simulink model "Control_systemR2024a"  (R2025b)
settings: Solver=FixedStepAuto  StartTime=0.0  StopTime=5  FixedStep=0.01  RelTol=1e-3
values from neighbouring files (symbols this model uses):
  beta = [beta1, beta2, beta3, beta4]    [initialize_simulink.m]
  calMp = Adgsl10m1' * calM1 * Adgsl10m1    [initialize_simulink.m]
  lM = zeros(4)    [initialize_simulink.m]
  m4g = m4 * 9.81    (= 68.67)    [initialize_simulink.m]
  xi = [xi1, xi2, xi3, xi4]    [initialize_simulink.m]
settings Model: Creator=81135  LastModifiedBy=dixiao

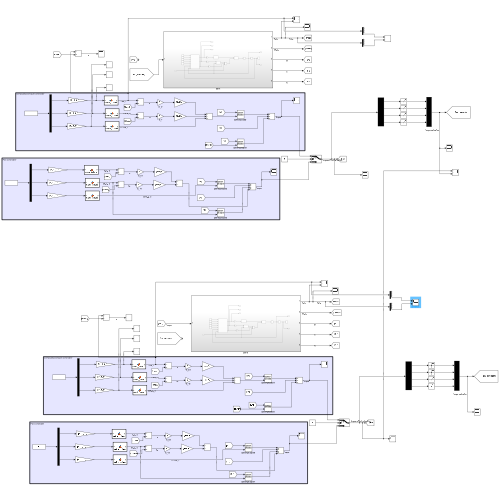
[thumbnail: Simulink's stored preview of the top-level diagram]
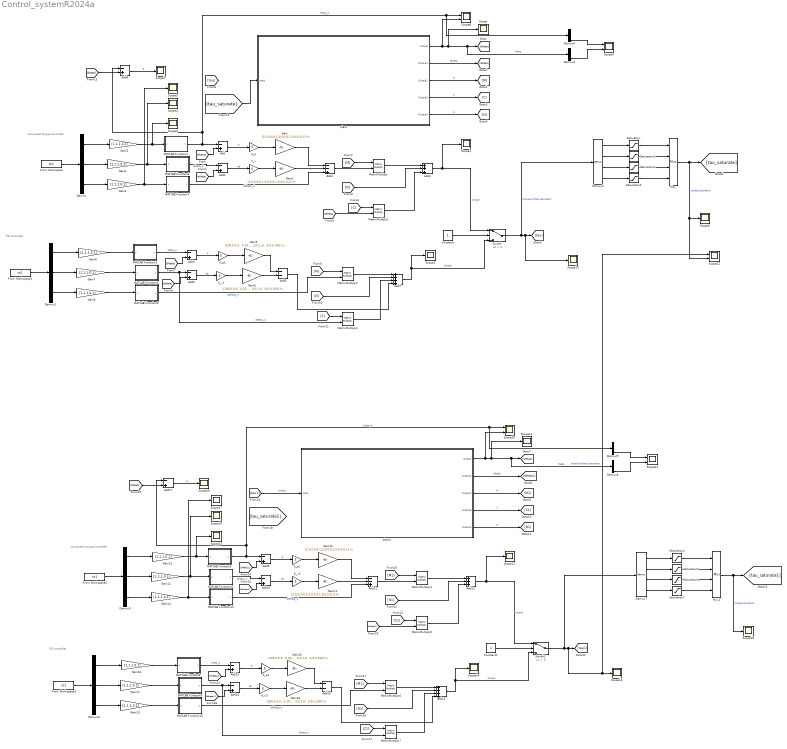
== system Control_systemR2024a ==
  note: PD controller
  note: computed torque controller
  note: computed torque controller
  note: PD controller
  Add{,1,4..5,8..10,13..14,17} (10 alike) : Sum  Inputs=-+
  Add11 : Sum  Inputs=--+
  Add12 : Sum  Inputs=+++
  Add15 : Sum  Inputs=--
  Add16 : Sum  Inputs=++++
  Add2 : Sum  Inputs=--+
  Add3 : Sum  Inputs=+++
  Add6 : Sum  Inputs=--
  Add7 : Sum  Inputs=++++
  Constant : Constant
  Constant1 : Constant
  Demux{,1,5..6} (4 alike) : Demux  Outputs=3
  Demux{2..4,7..9} (6 alike) : Demux
  From Workspace{,1..3} (4 alike) : FromWorkspace  VariableName=ts1
  Gain{,1,10..11} (4 alike) : Gain  Gain=[1,0,0,0;0,1,0,0;0,0,1,0;0,0,0,1]  Multiplication=Matrix(K*u)
  Gain{2..4,7..9,12..14,17..19} (12 alike) : Gain  Gain=[1,1,1,0.1]
  Gain{5..6,15..16} (4 alike) : Gain  Gain="[100,0,0,0;  0,100,0,0;  0,0,1,0;  0,0,0,100]"  Multiplication=Matrix(K*u)
  K_p{,1..3} (4 alike) : Gain  Gain=5
  K_v{,1..3} (4 alike) : Gain  Gain=5
  MATLAB Function1 : MATLAB Function  TreatAsAtomicUnit=on
  MATLAB Function10 : MATLAB Function  TreatAsAtomicUnit=on
  MATLAB Function11 : MATLAB Function  TreatAsAtomicUnit=on
  MATLAB Function12 : MATLAB Function  TreatAsAtomicUnit=on
  MATLAB Function2 : MATLAB Function  TreatAsAtomicUnit=on
  MATLAB Function3 : MATLAB Function  TreatAsAtomicUnit=on
  MATLAB Function4 : MATLAB Function  TreatAsAtomicUnit=on
  MATLAB Function5 : MATLAB Function  TreatAsAtomicUnit=on
  MATLAB Function6 : MATLAB Function  TreatAsAtomicUnit=on
  MATLAB Function7 : MATLAB Function  TreatAsAtomicUnit=on
  MATLAB Function8 : MATLAB Function  TreatAsAtomicUnit=on
  MATLAB Function9 : MATLAB Function  TreatAsAtomicUnit=on
  MatrixMultiply{,1..7} (8 alike) : Product  Multiplication=Matrix(*)
  Mux : Mux
  Mux1 : Mux
  Saturation : Saturate  UpperLimit=2000  LowerLimit=-2000
  Saturation{1..2,5..6} (4 alike) : Saturate  UpperLimit=1000  LowerLimit=-1000
  Saturation3 : Saturate  UpperLimit=100  LowerLimit=-100
  Saturation4 : Saturate  UpperLimit=2000  LowerLimit=-2000
  Saturation7 : Saturate  UpperLimit=100  LowerLimit=-100
  Scope{,1..7,10..19} (18 alike) : Scope
      Scope settings: ActiveDisplayYMinimum=-0.45551  ActiveDisplayYMaximum=2.83276
      Scope1 settings: ActiveDisplayYMinimum=-5169.19127  ActiveDisplayYMaximum=5422.5513  DataLoggingVariableName=ScopeData3
      Scope10 settings: ActiveDisplayYMinimum=-2408.79583  ActiveDisplayYMaximum=5518.79264  DataLoggingVariableName=ScopeData4
      Scope11 settings: ActiveDisplayYMinimum=-0.45551  ActiveDisplayYMaximum=2.83276  DataLoggingVariableName=ScopeData5
      Scope12 settings: ActiveDisplayYMinimum=-5169.19127  ActiveDisplayYMaximum=5422.5513  DataLoggingVariableName=ScopeData6
      Scope13 settings: ActiveDisplayYMinimum=-5240.02366  ActiveDisplayYMaximum=5364.1419  DataLoggingVariableName=ScopeData7
      Scope14 settings: ActiveDisplayYMinimum=-5091.129  ActiveDisplayYMaximum=5351.713  DataLoggingVariableName=ScopeData8
      Scope15 settings: ActiveDisplayYMinimum=-0.125  ActiveDisplayYMaximum=1.125  DataLoggingVariableName=ScopeData9
      Scope16 settings: ActiveDisplayYMinimum=-0.41667  ActiveDisplayYMaximum=3.75  DataLoggingVariableName=ScopeData10
      Scope17 settings: ActiveDisplayYMinimum=-41.66667  ActiveDisplayYMaximum=41.66667  DataLoggingVariableName=ScopeData11
      Scope18 settings: ActiveDisplayYMinimum=-2500  ActiveDisplayYMaximum=2500  DataLoggingVariableName=ScopeData12
      Scope19 settings: ActiveDisplayYMinimum=-0.0046  ActiveDisplayYMaximum=0.04138  DataLoggingVariableName=ScopeData13
      Scope2 settings: ActiveDisplayYMinimum=-5091.129  ActiveDisplayYMaximum=5351.713  DataLoggingVariableName=ScopeData2
      Scope3 settings: ActiveDisplayYMinimum=-0.125  ActiveDisplayYMaximum=1.125  DataLoggingVariableName=ScopeData4
      Scope4 settings: ActiveDisplayYMinimum=-0.41667  ActiveDisplayYMaximum=3.75  DataLoggingVariableName=ScopeData5
      Scope5 settings: ActiveDisplayYMinimum=-41.66667  ActiveDisplayYMaximum=41.66667  DataLoggingVariableName=ScopeData6
      Scope6 settings: ActiveDisplayYMinimum=-2500  ActiveDisplayYMaximum=2500  DataLoggingVariableName=ScopeData7
      Scope7 settings: ActiveDisplayYMinimum=-1.1474  ActiveDisplayYMaximum=1.79852
  Scope{8..9,20..22} (5 alike) : Scope  NumInputPorts=2
      Scope20 settings: ActiveDisplayYMinimum=-0.1296  ActiveDisplayYMaximum=1.16638  DataLoggingVariableName=ScopeData14
      Scope21 settings: ActiveDisplayYMinimum=-0.01253  ActiveDisplayYMaximum=0.11281  DataLoggingVariableName=ScopeData15
      Scope22 settings: ActiveDisplayYMinimum=1.92293  ActiveDisplayYMaximum=75.33497  DataLoggingVariableName=ScopeData16
      Scope8 settings: ActiveDisplayYMinimum=-1.3690570459134255  ActiveDisplayYMaximum=2.8522624254214288  DataLoggingVariableName=ScopeData2
      Scope9 settings: ActiveDisplayYMinimum=-0.01253  ActiveDisplayYMaximum=0.11281  DataLoggingVariableName=ScopeData3
  Switch : Switch  Criteria=u2 > Threshold  SaturateOnIntegerOverflow=off  InputSameDT=off
  Switch1 : Switch  Criteria=u2 > Threshold  SaturateOnIntegerOverflow=off  InputSameDT=off
  plant : Subsystem
  plant1 : Subsystem
  wires:
  plant/1(Output) -> Scope8/2, Demux3/1, [theta], Scope/1  "theta"
  plant/2(Output1) -> [dtheta]  "dtheta"
  plant/3(Output2) -> [M]  "M"
  plant/4(Output3) -> [C]  "C"
  plant/5(Output4) -> [N]  "N"
  Add/1 -> K_p/1  "e"
  [dtheta] -> MatrixMultiply1/2
  MatrixMultiply/1 -> Add3/1
  Gain1/1 -> Add2/2
  Demux/2 -> Gain2/1
  [N] -> Add3/2
  From Workspace/1 -> Demux/1
  [theta] -> Add/2
  Add1/1 -> K_v/1  "de"
  MATLAB Function6/1(y) -> Add1/1  "dtheta_d"
  [M] -> MatrixMultiply/1
  [dtheta] -> Add1/2
  Add3/1 -> Switch/1, Scope1/1  "torque"
  [C] -> MatrixMultiply1/1
  Add2/1 -> MatrixMultiply/2
  MATLAB Function7/1(y) -> Add2/3  "ddtheta_d"
  MatrixMultiply1/1 -> Add3/3
  Gain/1 -> Add2/1
  Demux/1 -> Gain3/1
  MATLAB Function1/1(y) -> Demux4/1, Scope8/1, Add8/1, Add/1  "theta_d"
  Gain4/1 -> Scope5/1, MATLAB Function7/1(u)
  Gain2/1 -> Scope4/1, MATLAB Function6/1(u)
  Gain3/1 -> Scope3/1, MATLAB Function1/1(u)
  K_v/1 -> Gain1/1
  K_p/1 -> Gain/1
  Demux/3 -> Gain4/1
  [N] -> Add7/2
  Demux1/2 -> Gain7/1
  Gain6/1 -> Add6/2
  Add4/1 -> K_p1/1  "e"
  [C] -> MatrixMultiply3/1
  Add7/1 -> Switch/3, Scope2/1  "torque"
  MatrixMultiply3/1 -> Add7/3
  Gain5/1 -> Add6/1
  MATLAB Function4/1(y) -> MatrixMultiply2/2  "ddtheta_d"
  Demux1/1 -> Gain8/1
  Gain9/1 -> MATLAB Function4/1(u)
  Gain8/1 -> MATLAB Function2/1(u)
  Gain7/1 -> MATLAB Function3/1(u)
  MATLAB Function2/1(y) -> Add4/1  "theta_d"
  From Workspace1/1 -> Demux1/1
  MatrixMultiply2/1 -> Add7/1
  Demux1/3 -> Gain9/1
  K_v1/1 -> Gain6/1
  [M] -> MatrixMultiply2/1
  MATLAB Function3/1(y) -> MatrixMultiply3/2, Add5/1  "dtheta_d"
  [dtheta] -> Add5/2
  Add5/1 -> K_v1/1  "de"
  K_p1/1 -> Gain5/1
  [theta] -> Add4/2
  Add6/1 -> Add7/4
  Constant/1 -> Switch/2
  Demux2/4 -> Saturation3/1
  Demux2/2 -> Saturation1/1
  Demux2/1 -> Saturation/1
  Demux2/3 -> Saturation2/1
  Switch/1 -> Demux2/1, Scope10/1, [tau]  "torque without saturation"
  Saturation/1 -> Mux/1
  Saturation1/1 -> Mux/2
  Saturation2/1 -> Mux/3
  Saturation3/1 -> Mux/4
  Mux/1 -> Scope22/2, Scope6/1, [tau_saturate]  "torque saturation"
  [theta] -> Add8/2
  Add8/1 -> Scope7/1  "e"
  Demux4/4 -> Scope9/1
  Demux3/4 -> Scope9/2
  [theta1] -> Add17/2
  Add17/1 -> Scope19/1  "e"
  Demux9/4 -> Scope21/1
  Saturation6/1 -> Mux1/3
  Add9/1 -> K_p2/1  "e"
  Gain16/1 -> Add15/2
  Saturation5/1 -> Mux1/2
  MATLAB Function5/1(y) -> Demux9/1, Scope20/1, Add17/1, Add9/1  "theta_d"
  [C1] -> MatrixMultiply7/1
  Gain17/1 -> MATLAB Function9/1(u)
  MATLAB Function10/1(y) -> MatrixMultiply6/2  "ddtheta_d"
  Saturation4/1 -> Mux1/1
  Switch1/1 -> Demux7/1, Scope22/1, Scope13/1, [tau1]  "torque without saturation"
  Mux1/1 -> Scope18/1, [tau_saturate1]  "torque saturation"
  Saturation7/1 -> Mux1/4
  MATLAB Function12/1(y) -> Add11/3  "ddtheta_d"
  [dtheta1] -> Add10/2
  MATLAB Function8/1(y) -> Add13/1  "theta_d"
  [theta1] -> Add9/2
  plant1/3(Output2) -> [M1]  "M"
  [dtheta1] -> Add14/2
  plant1/2(Output1) -> [dtheta1]  "dtheta"
  Demux7/1 -> Saturation4/1
  MatrixMultiply6/1 -> Add16/1
  Gain10/1 -> Add11/1
  Demux6/1 -> Gain18/1
  From Workspace2/1 -> Demux5/1
  Add15/1 -> Add16/4
  K_p3/1 -> Gain15/1
  Gain15/1 -> Add15/1
  [M1] -> MatrixMultiply6/1
  Demux6/3 -> Gain19/1
  plant1/1(Output) -> Scope20/2, Demux8/1, [theta1], Scope11/1  "theta"
  Add14/1 -> K_v3/1  "de"
  K_v2/1 -> Gain11/1
  MatrixMultiply7/1 -> Add16/3
  Demux8/4 -> Scope21/2
  K_v3/1 -> Gain16/1
  [N1] -> Add16/2
  Demux5/3 -> Gain14/1
  Gain12/1 -> Scope16/1, MATLAB Function11/1(u)
  [dtheta1] -> MatrixMultiply5/2
  [tau1] -> plant1/1(Input)  "torque"
  Constant1/1 -> Switch1/2
  K_p2/1 -> Gain10/1
  Gain19/1 -> MATLAB Function10/1(u)
  Gain13/1 -> Scope15/1, MATLAB Function5/1(u)
  plant1/4(Output3) -> [C1]  "C"
  Demux7/4 -> Saturation7/1
  Add16/1 -> Switch1/3, Scope14/1  "torque"
  MatrixMultiply4/1 -> Add12/1
  MATLAB Function11/1(y) -> Add10/1  "dtheta_d"
  Add12/1 -> Switch1/1, Scope12/1  "torque"
  Demux5/2 -> Gain12/1
  [C1] -> MatrixMultiply5/1
  Gain18/1 -> MATLAB Function8/1(u)
  [M1] -> MatrixMultiply4/1
  Demux5/1 -> Gain13/1
  MATLAB Function9/1(y) -> MatrixMultiply7/2, Add14/1  "dtheta_d"
  From Workspace3/1 -> Demux6/1
  [theta1] -> Add13/2
  Add10/1 -> K_v2/1  "de"
  MatrixMultiply5/1 -> Add12/3
  Demux7/2 -> Saturation5/1
  Add11/1 -> MatrixMultiply4/2
  Gain14/1 -> Scope17/1, MATLAB Function12/1(u)
  Demux7/3 -> Saturation6/1
  Gain11/1 -> Add11/2
  Demux6/2 -> Gain17/1
  [N1] -> Add12/2
  plant1/5(Output4) -> [N1]  "N"
  Add13/1 -> K_p3/1  "e"
  [tau_saturate] -> plant/1(Input)

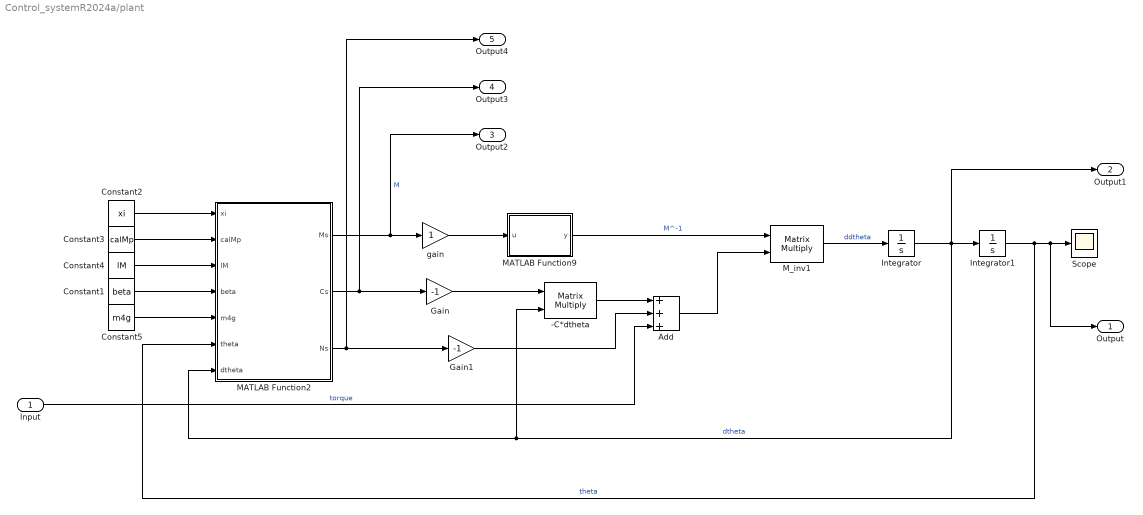
== system Control_systemR2024a/plant ==
  Input : Inport
  -C*dtheta : Product  Multiplication=Matrix(*)
  Add : Sum  Inputs=+++
  Constant1 : Constant  Value=beta
  Constant2 : Constant  Value=xi
  Constant3 : Constant  Value=calMp
  Constant4 : Constant  Value=lM
  Constant5 : Constant  Value=m4g
  Gain : Gain  Gain=-1
  Gain1 : Gain  Gain=-1
  Integrator : Integrator  InitialCondition=[0;0;0;0]
  Integrator1 : Integrator  InitialCondition=[0;0;0;0]
  MATLAB Function2 : MATLAB Function  TreatAsAtomicUnit=on
  MATLAB Function9 : MATLAB Function  TreatAsAtomicUnit=on
  M_inv1 : Product  Multiplication=Matrix(*)
  Scope : Scope
      settings: ActiveDisplayYMinimum=-0.13004  ActiveDisplayYMaximum=1.17037
  gain : Gain
  Output : Outport
  Output1 : Outport  Port=2
  Output2 : Outport  Port=3
  Output3 : Outport  Port=4
  Output4 : Outport  Port=5
  wires:
  MATLAB Function2/1(Ms) -> Output2/1, gain/1  "M"
  Integrator/1 -> Output1/1, -C*dtheta/2, MATLAB Function2/7(dtheta), Integrator1/1  "dtheta"
  Gain/1 -> -C*dtheta/1
  Constant4/1 -> MATLAB Function2/3(lM)
  -C*dtheta/1 -> Add/1
  Constant3/1 -> MATLAB Function2/2(calMp)
  Integrator1/1 -> MATLAB Function2/6(theta), Output/1, Scope/1  "theta"
  M_inv1/1 -> Integrator/1  "ddtheta"
  MATLAB Function2/3(Ns) -> Output4/1, Gain1/1
  Constant1/1 -> MATLAB Function2/4(beta)
  Gain1/1 -> Add/2
  Constant5/1 -> MATLAB Function2/5(m4g)
  gain/1 -> MATLAB Function9/1(u)
  MATLAB Function2/2(Cs) -> Output3/1, Gain/1
  Constant2/1 -> MATLAB Function2/1(xi)
  Add/1 -> M_inv1/2
  MATLAB Function9/1(y) -> M_inv1/1  "M^-1"
  Input/1 -> Add/3  "torque"

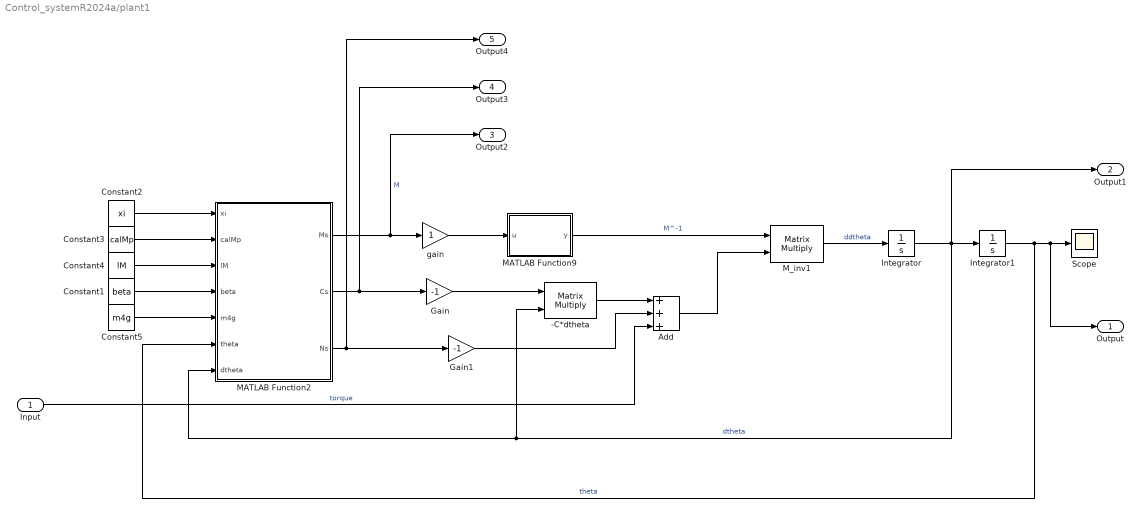
== system Control_systemR2024a/plant1 ==
  Input : Inport
  -C*dtheta : Product  Multiplication=Matrix(*)
  Add : Sum  Inputs=+++
  Constant1 : Constant  Value=beta
  Constant2 : Constant  Value=xi
  Constant3 : Constant  Value=calMp
  Constant4 : Constant  Value=lM
  Constant5 : Constant  Value=m4g
  Gain : Gain  Gain=-1
  Gain1 : Gain  Gain=-1
  Integrator : Integrator  InitialCondition=[0;0;0;0]
  Integrator1 : Integrator  InitialCondition=[0;0;0;0]
  MATLAB Function2 : MATLAB Function  TreatAsAtomicUnit=on
  MATLAB Function9 : MATLAB Function  TreatAsAtomicUnit=on
  M_inv1 : Product  Multiplication=Matrix(*)
  Scope : Scope
      settings: ActiveDisplayYMinimum=-0.13004  ActiveDisplayYMaximum=1.17037
  gain : Gain
  Output : Outport
  Output1 : Outport  Port=2
  Output2 : Outport  Port=3
  Output3 : Outport  Port=4
  Output4 : Outport  Port=5
  wires:
  MATLAB Function2/1(Ms) -> Output2/1, gain/1  "M"
  Integrator/1 -> Output1/1, -C*dtheta/2, MATLAB Function2/7(dtheta), Integrator1/1  "dtheta"
  Gain/1 -> -C*dtheta/1
  Constant4/1 -> MATLAB Function2/3(lM)
  -C*dtheta/1 -> Add/1
  Constant3/1 -> MATLAB Function2/2(calMp)
  Integrator1/1 -> MATLAB Function2/6(theta), Output/1, Scope/1  "theta"
  M_inv1/1 -> Integrator/1  "ddtheta"
  MATLAB Function2/3(Ns) -> Output4/1, Gain1/1
  Constant1/1 -> MATLAB Function2/4(beta)
  Gain1/1 -> Add/2
  Constant5/1 -> MATLAB Function2/5(m4g)
  gain/1 -> MATLAB Function9/1(u)
  MATLAB Function2/2(Cs) -> Output3/1, Gain/1
  Constant2/1 -> MATLAB Function2/1(xi)
  Add/1 -> M_inv1/2
  MATLAB Function9/1(y) -> M_inv1/1  "M^-1"
  Input/1 -> Add/3  "torque"

== matlab function Control_systemR2024a/MATLAB Function5 ==
  data: u input; y output
function y = matrix_column(u)

    y = u(:);
end

== matlab function Control_systemR2024a/MATLAB Function8 ==
  data: u input; y output
function y = matrix_column(u)

    y = u(:);
end

== matlab function Control_systemR2024a/MATLAB Function9 ==
  data: u input; y output
function y = matrix_column(u)

    y = u(:);
end

== matlab function Control_systemR2024a/plant1/MATLAB Function2 ==
  data: xi input; Ms output; calMp input; lM input; beta input; m4g input; theta input; dtheta input; Cs output; Ns output
function [Ms,Cs,Ns] = MCNsim(xi,calMp,lM,beta,m4g,theta,dtheta)
    n = length(theta);
    Ms = zeros(n, n);
    Cs = zeros(n, n);
    % Ns = zeros(n, 1);
    
    % ========== 关键步骤1：预先计算所有需要的变换矩阵 g = exp(ξθ) ==========
    g = cell(1, n+1);
    g{1} = eye(4);
    for i = 1:n
        xi_i = xi(:, i);
        g_joint = expm(hat_se3(xi_i) * theta(i));
        g{i+1} = g{i} * g_joint;
    end
    
    % ========== 关键步骤2：计算所有 A_{ij} ==========
    A = cell(n, n);
    for i = 1:n
        for j = 1:n
            if i > j
                g_ji = inv(g{j+1}) * g{i+1};
                A{i,j} = inv(adjmg(g_ji));
            elseif i == j
                A{i,j} = eye(6);
            else
                A{i,j} = zeros(6);
            end
        end
    end
    
    % ========== 步骤3：计算惯性矩阵 M ==========
    for i = 1:n
        for j = 1:n
            M_ij = 0;
            for l = lM(i, j):n
                M_l = calMp(1:6, 1:6, l);
                term = xi(:, i)' * A{l, i}' * M_l * A{l, j} * xi(:, j);
                M_ij = M_ij + term;
            end
            Ms(i, j) = M_ij;
        end
    end
    
    % ========== 步骤4：计算科氏矩阵 C（解析公式） ==========
    for i = 1:n
        for j = 1:n
            C_ij = 0;
            for k = 1:n
                dM_ij_dtheta_k = compute_partial_M(xi, calMp, lM, A, i, j, k, n);
                dM_ik_dtheta_j = compute_partial_M(xi, calMp, lM, A, i, k, j, n);
                dM_kj_dtheta_i = compute_partial_M(xi, calMp, lM, A, k, j, i, n);
                C_ij = C_ij + 0.5 * (dM_ij_dtheta_k + dM_ik_dtheta_j - dM_kj_dtheta_i) * dtheta(k);
            end
            Cs(i, j) = C_ij;
        end
    end
    
    % ========== 步骤5：计算 N（根据图片公式和你的物理参数） ==========
    % 公式：N_i = ∂V/∂θ_i + β_i * θ̇_i
    
    % 5.1 计算重力势能梯度 ∂V/∂θ_i
    grad_V = compute_gravity_potential_gradient(xi, calMp, g, n);
    
    % 5.2 计算粘性摩擦项 β_i * θ̇_i 
    % 你的beta是向量: [beta1, beta2, beta3, beta4]，单位对应各关节类型
    friction_term = beta(:) .* dtheta(:); % 确保维度匹配
    
    % 5.3 计算总N项: N = ∂V/∂θ + β * θ̇
    Ns = -grad_V + friction_term;
end

% ========== 辅助函数：计算重力势能梯度 ∂V/∂θ (已根据你的代码调整) ==========
function grad_V = compute_gravity_potential_gradient(xi, calMp, g, n)
    % 计算重力势能 V(θ) 关于 θ 的梯度
    % 根据旋量理论：∂V/∂θ_i = Σ_{l=i}^n ξ_i^T * (Ad^{-1}(g_{0l}))^T * M_l * G_0
    % 其中 G_0 是基座标系下的重力旋量
    
    grad_V = zeros(n, 1);
    
    % 基座标系下的重力加速度向量 (沿负z轴，大小9.81 m/s²)
    % 注意：重力对旋量的贡献取决于表示法
    % 对于空间旋量 ξ = [v; ω]，重力旋量为 G = [0; -g]
    g_accel = [0; 0; -9.81]; % 重力加速度向量
    
    % 构造基座标系下的重力旋量 G_0
    % 根据你的旋量构造方式 (xi = [-hat(w)*q; w])，这是空间旋量表示
    % 对于空间旋量，重力只有线速度部分：G_0 = [-g_accel; 0]
    G_base = zeros(6, 1);
    G_base(1:3) = -g_accel; % 线速度部分：负重力加速度
    G_base(4:6) = zeros(3,1); % 角速度部分：0
    
    for i = 1:n
        sum_term = 0;
        for l = i:n
            % 连杆 l 的空间惯性矩阵 (已在空间坐标系下，通过伴随变换得到)
            M_l = calMp(1:6, 1:6, l);
            
            % 从基座到连杆 l 的变换矩阵 g_{0l}
            g_0l = g{l+1};
            
            % 计算 Ad^{-1}(g_{0l}) 的转置
            Ad_inv = inv(adjmg(g_0l));
            Ad_inv_T = Ad_inv';
            
            % 计算该项对梯度 ∂V/∂θ_i 的贡献
            % 根据旋量理论，这是重力在关节i方向产生的广义力
            contribution = xi(:, i)' * Ad_inv_T * M_l * G_base;
            sum_term = sum_term + contribution;
        end
        
        % 得到的 sum_term 实际上是重力矩 G_i = -∂V/∂θ_i
        % 因此势能梯度为 ∂V/∂θ_i = -sum_term
        grad_V(i) = -sum_term;
    end
end

% ========== 其他辅助函数保持不变 ==========
function dM_ij_dtheta_k = compute_partial_M(xi, calMp, lM, A, i, j, k, n)
    dM_ij_dtheta_k = 0;
    
    for l = lM(i, j):n
        M_l = calMp(1:6, 1:6, l);
        xi_i = xi(:, i);
        xi_j = xi(:, j);
        xi_k = xi(:, k);
        
        if k <= l
            % 计算 ad(A_{ki} * xi_i)
            A_ki_xi_i = A{k, i} * xi_i;
            ad_Aki_xi_i = adjoint_lie_algebra(A_ki_xi_i);
            
            % 计算 ad(A_{kj} * xi_j)
            A_kj_xi_j = A{k, j} * xi_j;
            ad_Akj_xi_j = adjoint_lie_algebra(A_kj_xi_j);
            
            term1 = (ad_Aki_xi_i * xi_k)' * A{l, k}' * M_l * A{l, j} * xi_j;
            term2 = xi_i' * A{l, i}' * M_l * A{l, k} * (ad_Akj_xi_j * xi_k);
            
            dM_ij_dtheta_k = dM_ij_dtheta_k + term1 + term2;
        end
    end
end

function ad_xi = adjoint_lie_algebra(xi)
    v = xi(1:3);
    w = xi(4:6);
    w_hat = hatm_num(w);
    v_hat = hatm_num(v);
    ad_xi = [w_hat, v_hat;
             zeros(3), w_hat];
end

function se3 = hat_se3(xi)
    v = xi(1:3);
    w = xi(4:6);
    se3 = [hatm_num(w), v;
           zeros(1,3), 0];
end

== matlab function Control_systemR2024a/plant1/MATLAB Function9 ==
  data: u input; y output
function y = matrix_inv(u)

    y = inv(u);
end

== matlab function Control_systemR2024a/MATLAB Function2 ==
  data: u input; y output
function y = matrix_column(u)

    y = u(:);
end

== matlab function Control_systemR2024a/plant/MATLAB Function2 ==
  data: xi input; Ms output; calMp input; lM input; beta input; m4g input; theta input; dtheta input; Cs output; Ns output
function [Ms,Cs,Ns] = MCNsim(xi,calMp,lM,beta,m4g,theta,dtheta)
    n = length(theta);
    Ms = zeros(n, n);
    Cs = zeros(n, n);
    % Ns = zeros(n, 1);
    
    % ========== 关键步骤1：预先计算所有需要的变换矩阵 g = exp(ξθ) ==========
    g = cell(1, n+1);
    g{1} = eye(4);
    for i = 1:n
        xi_i = xi(:, i);
        g_joint = expm(hat_se3(xi_i) * theta(i));
        g{i+1} = g{i} * g_joint;
    end
    
    % ========== 关键步骤2：计算所有 A_{ij} ==========
    A = cell(n, n);
    for i = 1:n
        for j = 1:n
            if i > j
                g_ji = inv(g{j+1}) * g{i+1};
                A{i,j} = inv(adjmg(g_ji));
            elseif i == j
                A{i,j} = eye(6);
            else
                A{i,j} = zeros(6);
            end
        end
    end
    
    % ========== 步骤3：计算惯性矩阵 M ==========
    for i = 1:n
        for j = 1:n
            M_ij = 0;
            for l = lM(i, j):n
                M_l = calMp(1:6, 1:6, l);
                term = xi(:, i)' * A{l, i}' * M_l * A{l, j} * xi(:, j);
                M_ij = M_ij + term;
            end
            Ms(i, j) = M_ij;
        end
    end
    
    % ========== 步骤4：计算科氏矩阵 C（解析公式） ==========
    for i = 1:n
        for j = 1:n
            C_ij = 0;
            for k = 1:n
                dM_ij_dtheta_k = compute_partial_M(xi, calMp, lM, A, i, j, k, n);
                dM_ik_dtheta_j = compute_partial_M(xi, calMp, lM, A, i, k, j, n);
                dM_kj_dtheta_i = compute_partial_M(xi, calMp, lM, A, k, j, i, n);
                C_ij = C_ij + 0.5 * (dM_ij_dtheta_k + dM_ik_dtheta_j - dM_kj_dtheta_i) * dtheta(k);
            end
            Cs(i, j) = C_ij;
        end
    end
    
    % ========== 步骤5：计算 N（根据图片公式和你的物理参数） ==========
    % 公式：N_i = ∂V/∂θ_i + β_i * θ̇_i
    
    % 5.1 计算重力势能梯度 ∂V/∂θ_i
    grad_V = compute_gravity_potential_gradient(xi, calMp, g, n);
    
    % 5.2 计算粘性摩擦项 β_i * θ̇_i 
    % 你的beta是向量: [beta1, beta2, beta3, beta4]，单位对应各关节类型
    friction_term = beta(:) .* dtheta(:); % 确保维度匹配
    
    % 5.3 计算总N项: N = ∂V/∂θ + β * θ̇
    Ns = -grad_V + friction_term;
end

% ========== 辅助函数：计算重力势能梯度 ∂V/∂θ (已根据你的代码调整) ==========
function grad_V = compute_gravity_potential_gradient(xi, calMp, g, n)
    % 计算重力势能 V(θ) 关于 θ 的梯度
    % 根据旋量理论：∂V/∂θ_i = Σ_{l=i}^n ξ_i^T * (Ad^{-1}(g_{0l}))^T * M_l * G_0
    % 其中 G_0 是基座标系下的重力旋量
    
    grad_V = zeros(n, 1);
    
    % 基座标系下的重力加速度向量 (沿负z轴，大小9.81 m/s²)
    % 注意：重力对旋量的贡献取决于表示法
    % 对于空间旋量 ξ = [v; ω]，重力旋量为 G = [0; -g]
    g_accel = [0; 0; -9.81]; % 重力加速度向量
    
    % 构造基座标系下的重力旋量 G_0
    % 根据你的旋量构造方式 (xi = [-hat(w)*q; w])，这是空间旋量表示
    % 对于空间旋量，重力只有线速度部分：G_0 = [-g_accel; 0]
    G_base = zeros(6, 1);
    G_base(1:3) = -g_accel; % 线速度部分：负重力加速度
    G_base(4:6) = zeros(3,1); % 角速度部分：0
    
    for i = 1:n
        sum_term = 0;
        for l = i:n
            % 连杆 l 的空间惯性矩阵 (已在空间坐标系下，通过伴随变换得到)
            M_l = calMp(1:6, 1:6, l);
            
            % 从基座到连杆 l 的变换矩阵 g_{0l}
            g_0l = g{l+1};
            
            % 计算 Ad^{-1}(g_{0l}) 的转置
            Ad_inv = inv(adjmg(g_0l));
            Ad_inv_T = Ad_inv';
            
            % 计算该项对梯度 ∂V/∂θ_i 的贡献
            % 根据旋量理论，这是重力在关节i方向产生的广义力
            contribution = xi(:, i)' * Ad_inv_T * M_l * G_base;
            sum_term = sum_term + contribution;
        end
        
        % 得到的 sum_term 实际上是重力矩 G_i = -∂V/∂θ_i
        % 因此势能梯度为 ∂V/∂θ_i = -sum_term
        grad_V(i) = -sum_term;
    end
end

% ========== 其他辅助函数保持不变 ==========
function dM_ij_dtheta_k = compute_partial_M(xi, calMp, lM, A, i, j, k, n)
    dM_ij_dtheta_k = 0;
    
    for l = lM(i, j):n
        M_l = calMp(1:6, 1:6, l);
        xi_i = xi(:, i);
        xi_j = xi(:, j);
        xi_k = xi(:, k);
        
        if k <= l
            % 计算 ad(A_{ki} * xi_i)
            A_ki_xi_i = A{k, i} * xi_i;
            ad_Aki_xi_i = adjoint_lie_algebra(A_ki_xi_i);
            
            % 计算 ad(A_{kj} * xi_j)
            A_kj_xi_j = A{k, j} * xi_j;
            ad_Akj_xi_j = adjoint_lie_algebra(A_kj_xi_j);
            
            term1 = (ad_Aki_xi_i * xi_k)' * A{l, k}' * M_l * A{l, j} * xi_j;
            term2 = xi_i' * A{l, i}' * M_l * A{l, k} * (ad_Akj_xi_j * xi_k);
            
            dM_ij_dtheta_k = dM_ij_dtheta_k + term1 + term2;
        end
    end
end

function ad_xi = adjoint_lie_algebra(xi)
    v = xi(1:3);
    w = xi(4:6);
    w_hat = hatm_num(w);
    v_hat = hatm_num(v);
    ad_xi = [w_hat, v_hat;
             zeros(3), w_hat];
end

function se3 = hat_se3(xi)
    v = xi(1:3);
    w = xi(4:6);
    se3 = [hatm_num(w), v;
           zeros(1,3), 0];
end

== matlab function Control_systemR2024a/MATLAB Function1 ==
  data: u input; y output
function y = matrix_column(u)

    y = u(:);
end

== matlab function Control_systemR2024a/MATLAB Function6 ==
  data: u input; y output
function y = matrix_column(u)

    y = u(:);
end

== matlab function Control_systemR2024a/MATLAB Function7 ==
  data: u input; y output
function y= matrix_column(u)

    y = u(:);
end

== matlab function Control_systemR2024a/MATLAB Function3 ==
  data: u input; y output
function y = matrix_column(u)

    y = u(:);
end

== matlab function Control_systemR2024a/MATLAB Function4 ==
  data: u input; y output
function y= matrix_column(u)

    y = u(:);
end

== matlab function Control_systemR2024a/MATLAB Function10 ==
  data: u input; y output
function y= matrix_column(u)

    y = u(:);
end

== matlab function Control_systemR2024a/MATLAB Function11 ==
  data: u input; y output
function y = matrix_column(u)

    y = u(:);
end

== matlab function Control_systemR2024a/plant/MATLAB Function9 ==
  data: u input; y output
function y = matrix_inv(u)

    y = inv(u);
end

== matlab function Control_systemR2024a/MATLAB Function12 ==
  data: u input; y output
function y= matrix_column(u)

    y = u(:);
end
